simulink model "modelo_SAS"  (R2022b)
settings: Solver=VariableStepAuto  StartTime=0.0  StopTime=340  RelTol=1e-3
values from neighbouring files (symbols this model uses):
  LT = sist_lat(p)    [Solucion_Ecuaciones.m]    (also in pruebas.m)
libraries: cstblocks x4
settings Model: Creator=raulm  LastModifiedBy=VSPC
settings ModelReferenceCC: EnableRefExpFcnMdlSchedulingChecks=on

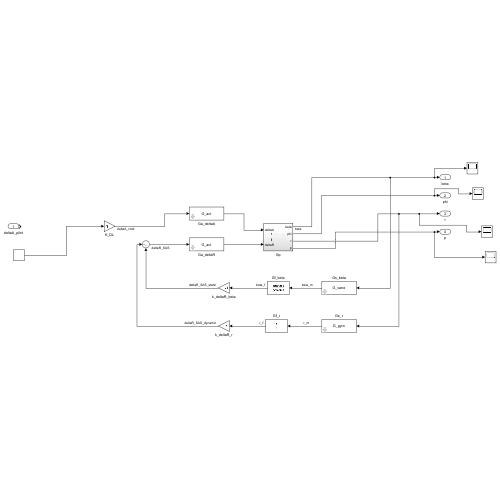
[thumbnail: Simulink's stored preview of the top-level diagram]
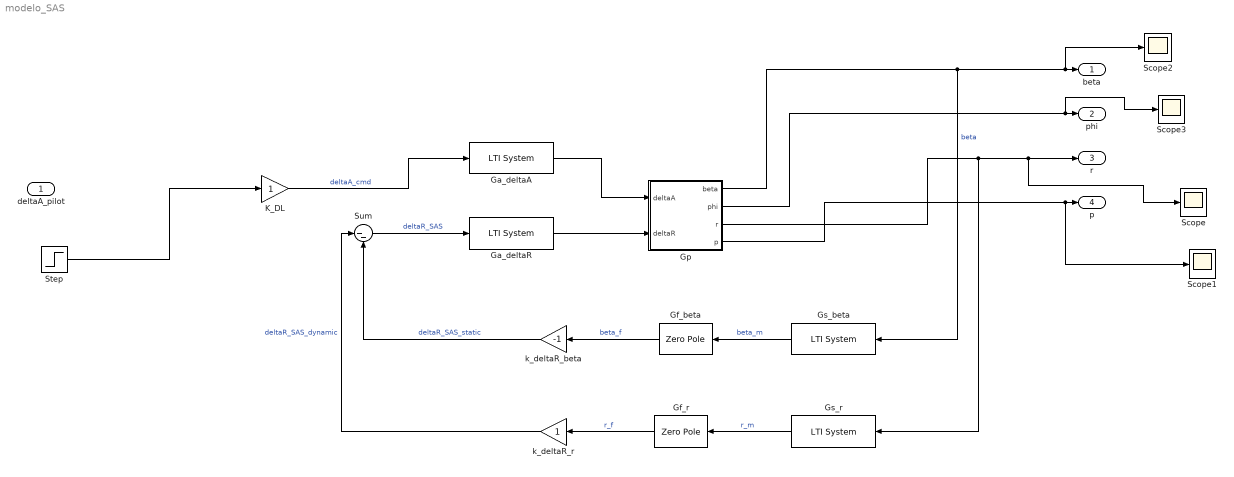
== system modelo_SAS ==
  deltaA_pilot : Inport
  Ga_deltaA : cstblocks/LTI System  sys=G_act  IC=[]
  Ga_deltaR : cstblocks/LTI System  sys=G_act  IC=[]
  Gf_beta : ZeroPole  Poles=[1]
  Gf_r : ZeroPole  Zeros=[0]  Poles=0  Gain=1
  Gp : Subsystem
  Gs_beta : cstblocks/LTI System  sys=G_vane  IC=[]
  Gs_r : cstblocks/LTI System  sys=G_gyro  IC=[]
  K_DL : Gain
  Scope{,1..3} (4 alike) : Scope
  Step : Step  SampleTime=0
  Sum : Sum  Inputs=|--
  k_deltaR_beta : Gain  Gain=-1
  k_deltaR_r : Gain
  beta : Outport
  phi : Outport  Port=2
  r : Outport  Port=3
  p : Outport  Port=4
  wires:
  Gp/3(r) -> Gs_r/1, Scope/1, r/1
  k_deltaR_r/1 -> Sum/1  "deltaR_SAS_dynamic"
  K_DL/1 -> Ga_deltaA/1  "deltaA_cmd"
  Gs_beta/1 -> Gf_beta/1  "beta_m"
  Gf_r/1 -> k_deltaR_r/1  "r_f"
  Gs_r/1 -> Gf_r/1  "r_m"
  Gf_beta/1 -> k_deltaR_beta/1  "beta_f"
  Ga_deltaR/1 -> Gp/2(deltaR)
  Sum/1 -> Ga_deltaR/1  "deltaR_SAS"
  Gp/2(phi) -> Scope3/1, phi/1
  Gp/1(beta) -> Gs_beta/1, Scope2/1, beta/1  "beta"
  Gp/4(p) -> Scope1/1, p/1
  k_deltaR_beta/1 -> Sum/2  "deltaR_SAS_static"
  Ga_deltaA/1 -> Gp/1(deltaA)
  Step/1 -> K_DL/1

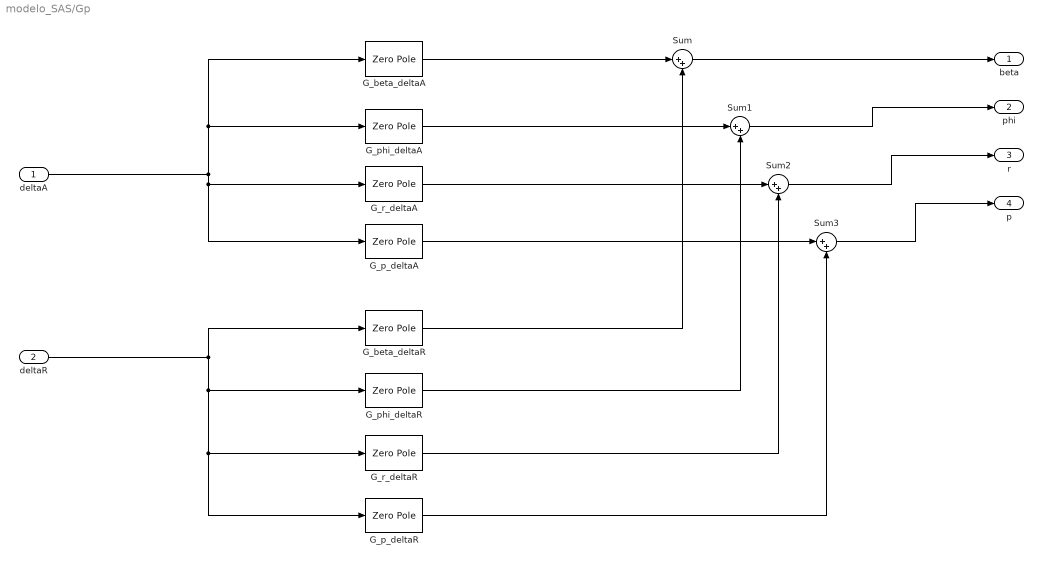
== system modelo_SAS/Gp ==
  deltaA : Inport
  deltaR : Inport  Port=2
  G_beta_deltaA : ZeroPole  Zeros=LT.FT_fact.FTdeltaA_beta.Z{1,1}  Poles=LT.FT_fact.FTdeltaA_beta.P{1,1}  Gain=LT.FT_fact.FTdeltaA_beta.K
  G_beta_deltaR : ZeroPole  Zeros=LT.FT_fact.FTdeltaR_beta.Z{1,1}  Poles=LT.FT_fact.FTdeltaR_beta.P{1,1}  Gain=LT.FT_fact.FTdeltaR_beta.K
  G_p_deltaA : ZeroPole  Zeros=LT.FT_fact.FTdeltaA_p.Z{1,1}  Poles=LT.FT_fact.FTdeltaA_p.P{1,1}  Gain=LT.FT_fact.FTdeltaA_p.K
  G_p_deltaR : ZeroPole  Zeros=LT.FT_fact.FTdeltaR_p.Z{1,1}  Poles=LT.FT_fact.FTdeltaR_p.P{1,1}  Gain=LT.FT_fact.FTdeltaR_p.K
  G_phi_deltaA : ZeroPole  Zeros=LT.FT_fact.FTdeltaA_phi.Z{1,1}  Poles=LT.FT_fact.FTdeltaA_phi.P{1,1}  Gain=LT.FT_fact.FTdeltaA_phi.K
  G_phi_deltaR : ZeroPole  Zeros=LT.FT_fact.FTdeltaR_phi.Z{1,1}  Poles=LT.FT_fact.FTdeltaR_phi.P{1,1}  Gain=LT.FT_fact.FTdeltaR_phi.K
  G_r_deltaA : ZeroPole  Zeros=LT.FT_fact.FTdeltaA_r.Z{1,1}  Poles=LT.FT_fact.FTdeltaA_r.P{1,1}  Gain=LT.FT_fact.FTdeltaA_r.K
  G_r_deltaR : ZeroPole  Zeros=LT.FT_fact.FTdeltaR_r.Z{1,1}  Poles=LT.FT_fact.FTdeltaR_r.P{1,1}  Gain=LT.FT_fact.FTdeltaR_r.K
  Sum{,1..3} (4 alike) : Sum  Inputs=|++
  beta : Outport
  phi : Outport  Port=2
  r : Outport  Port=3
  p : Outport  Port=4
  wires:
  deltaR/1 -> G_p_deltaR/1, G_r_deltaR/1, G_phi_deltaR/1, G_beta_deltaR/1
  G_phi_deltaA/1 -> Sum1/1
  deltaA/1 -> G_p_deltaA/1, G_r_deltaA/1, G_phi_deltaA/1, G_beta_deltaA/1
  G_r_deltaR/1 -> Sum2/2
  G_p_deltaA/1 -> Sum3/1
  G_r_deltaA/1 -> Sum2/1
  G_beta_deltaR/1 -> Sum/2
  Sum2/1 -> r/1
  Sum3/1 -> p/1
  Sum/1 -> beta/1
  G_p_deltaR/1 -> Sum3/2
  Sum1/1 -> phi/1
  G_beta_deltaA/1 -> Sum/1
  G_phi_deltaR/1 -> Sum1/2
